simulink model "plant"  (R2022a)
settings: Solver=VariableStepAuto  StartTime=0.0  StopTime=10.0  RelTol=1e-3
libraries: simulink x2
settings Model: Creator=Amirreza  LastModifiedBy=Amirreza

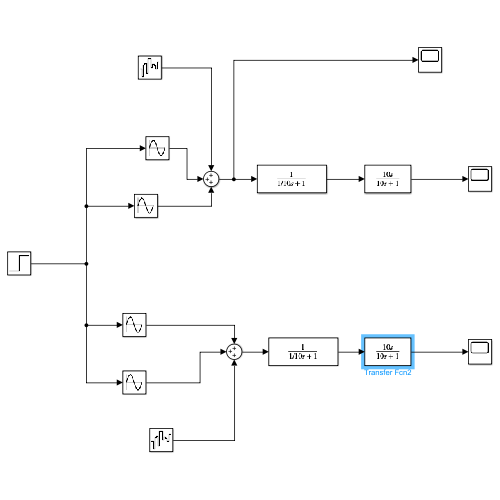
[thumbnail: Simulink's stored preview of the top-level diagram]
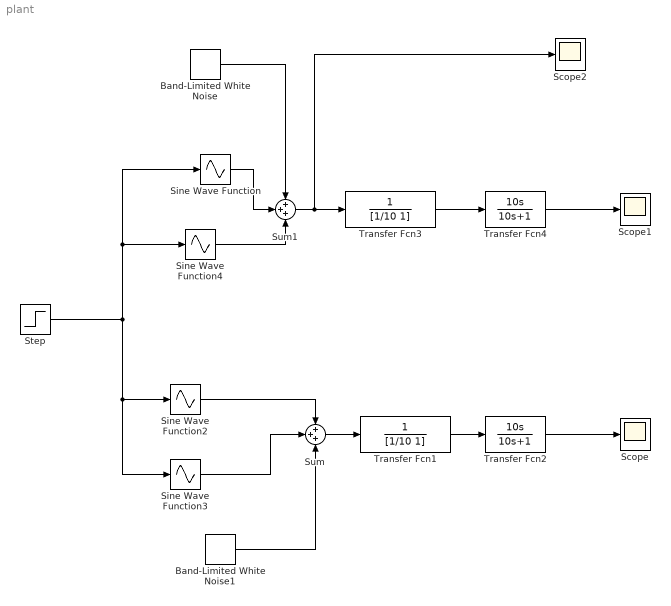
== system plant ==
  Band-Limited White Noise : simulink/Sources/Band-Limited White Noise  Cov=[0.1]  Ts=0.1  seed=[23341]
  Band-Limited White Noise1 : simulink/Sources/Band-Limited White Noise  Cov=[0.01]  Ts=0.1  seed=[23341]
  Scope : Scope
  Scope1 : Scope
  Scope2 : Scope
  Sine Wave Function : Sin  TimeSource=Use external signal  Amplitude=10  Frequency=2*pi  Phase=pi/2  SampleTime=0
  Sine Wave Function2 : Sin  TimeSource=Use external signal  Frequency=50*2*pi  SampleTime=0
  Sine Wave Function3 : Sin  TimeSource=Use external signal  Amplitude=0.1  Frequency=2*pi  SampleTime=0
  Sine Wave Function4 : Sin  TimeSource=Use external signal  Frequency=50*2*pi  SampleTime=0
  Step : Step  SampleTime=0
  Sum : Sum  Inputs=+++
  Sum1 : Sum  Inputs=+++
  Transfer Fcn1 : TransferFcn  Denominator=[1/10 1]
  Transfer Fcn2 : TransferFcn  Numerator=[10 0]  Denominator=[10 1]
  Transfer Fcn3 : TransferFcn  Denominator=[1/10 1]
  Transfer Fcn4 : TransferFcn  Numerator=[10 0]  Denominator=[10 1]
  wires:
  Step/1 -> Sine Wave Function4/1, Sine Wave Function/1, Sine Wave Function3/1, Sine Wave Function2/1
  Sine Wave Function2/1 -> Sum/1
  Sine Wave Function3/1 -> Sum/2
  Band-Limited White Noise1/1 -> Sum/3
  Sine Wave Function4/1 -> Sum1/3
  Sine Wave Function/1 -> Sum1/2
  Band-Limited White Noise/1 -> Sum1/1
  Sum1/1 -> Transfer Fcn3/1, Scope2/1
  Sum/1 -> Transfer Fcn1/1
  Transfer Fcn1/1 -> Transfer Fcn2/1
  Transfer Fcn2/1 -> Scope/1
  Transfer Fcn3/1 -> Transfer Fcn4/1
  Transfer Fcn4/1 -> Scope1/1
